simulink model "Pacemaker_group11_requirementtable"  (R2022a)
settings: Solver=FixedStepAuto  StartTime=0.0  StopTime=10.0  FixedStep=1e-3  RelTol=1e-3  EnableMultiTasking=on
undefined symbols (not defined in the file): A0, A1, D0, D1, D10, D11, D12, D13, D2, D3, D4, D5, D6, D7, D8, D9, magnitude, PTA0, PTA1, PTA2, PTB2, PTB23, PTB3, PTB9, PTC16, PTC17, PTC2, PTC3, PTC4, PTD0, PTD1, PTD2, PTD3
libraries: frdmk64flib x20, etargetslib x17, dspstat3 x1, simulink x1
(part 1 of 2)
settings Model: ExtModeTrigDuration=5  Creator=39200  LastModifiedBy=39200
settings OptimizationCC: EnhancedBackFolding=on  PassReuseOutputArgsAs=Individual arguments  ZeroExternalMemoryAtStartup=off  ZeroInternalMemoryAtStartup=off  MaxStackSize=64  OptimizeBlockOrder=speed  DifferentSizesBufferReuse=on  OptimizationCustomize=off  EfficientTunableParamExpr=on
settings DebuggingCC: ParameterTunabilityLossMsg=error
settings HardwareCC: ProdBitPerPointer=32  ProdBitPerSizeT=32  ProdBitPerPtrDiffT=32  ProdLargestAtomicInteger=Long  ProdLargestAtomicFloat=Double  ProdWordSize=32  ProdHWDeviceType=ARM Compatible->ARM Cortex
settings SFSimCC: MATLABDynamicMemAlloc=off
settings RTWCC: SystemTargetFile=ert.tlc  HardwareBoard=NXP FRDM-K64F  TLCOptions="-aInlineSetEventsForThisBaseRateFcn=TLC_FALSE -aSuppressMultiTaskScheduler=TLC_FALSE  -aRateBasedStepFcn=0"  TemplateMakefile=ert_default_tmf  Toolchain=GNU Tools for ARM Embedded Processors
settings CodeAppCC: ForceParamTrailComments=on  IgnoreCustomStorageClasses=off  OperatorAnnotations=on  SimulinkDataObjDesc=on  SFDataObjDesc=on  InsertBlockDesc=on
settings ERTTargetCC: ExtModeTransport=4  ExtModeMexFile=sendToCommService

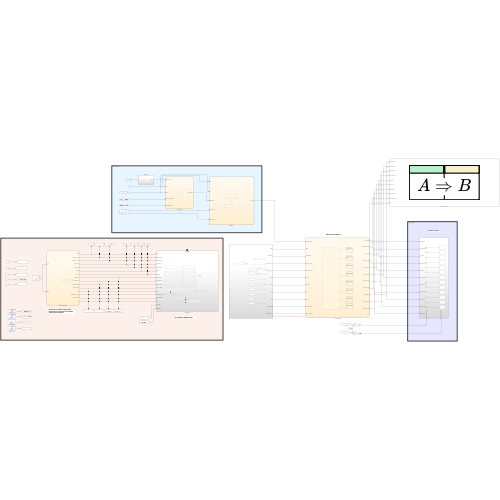
[thumbnail: Simulink's stored preview of the top-level diagram]
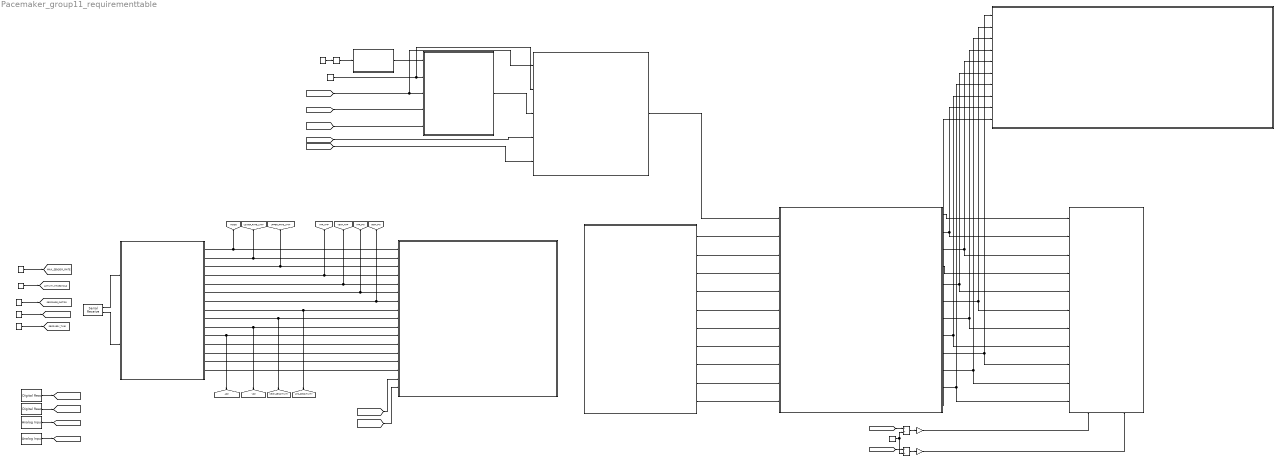
== system Pacemaker_group11_requirementtable ==
  note: Hardware Output
  note: Stateflow for All Modes
  note: Rate Modulation
  note: Stateflow for Initial Programmable Parameters and Input Programmable Parameters from DCM
  note: Inputs
  note: Send Data to DCM through UART
  note: Hardware Output
  ATR_SIGNAL : frdmk64flib/Analog Input  Whichpin=PTB2 (A0)  SampleTime=-1
  Acceleration1 : Subsystem
  Compare To Constant2 : simulink/Logic and Bit Operations/Compare To Constant  relop=>=  const=5  OutDataTypeStr=boolean
  Constant : Constant  Value=3.3
  Constant10 : Constant  Value=5
  Constant11 : Constant  Value=8
  Constant12 : Constant  Value=5
  Constant6 : Constant  Value=60
  Constant7 : Constant  Value=30
  Constant8 : Constant  Value=0.01
  Constant9 : Constant  Value=120
  Digital Read : frdmk64flib/Digital Read  Whichpin=PTC17 (D1)  SampleTime=-1
  Digital Read1 : frdmk64flib/Digital Read  Whichpin=PTC16 (D0)  SampleTime=-1
  Divide2 : Product  Inputs=*/
  Divide3 : Product  Inputs=*/
  Gain : Gain  Gain=100
  Gain1 : Gain  Gain=100
  Requirements Table : Requirements Table  TreatAsAtomicUnit=on
  Serial Communication1 : Stateflow chart  TreatAsAtomicUnit=on
      settings: PortSchema="{\"entries\":[{\"content\":{\"sides\":[{\"content\":{\"connectorIds\":[\"In1\",\"In2\"]},\"type\":\"ConnectorPlacement.EquallySpacedRectSide\",\"uuid\":\"901574a5-7e09-4852-8827-baac8e876273\"},{\"content\":{\"connectorIds\":[\"Out1\",\"Out2\",\"Out3\",\"Out4\",\"Out12\",\"Out5\",\"Out13\",\"Out14\",\"Out10\",\"Out6\",\"Out11\",\"Out7\",\"Out9\",\"Out8\",\"Out15\"],\"side\":\"RIGHT\"},\"type\":\"ConnectorPlacement.EquallySpacedRectSide\",\"uuid\":\"89d36c37-e833-4dfe-ae0b-2d9eccbce05b\"},{\"content\":{\"connectorIds\":[],\"side\":\"TOP\"},\"type\":\"ConnectorPlacement.EquallySpacedRectSide\",\"uuid\":\"eeb52db1-ccd5-49db-acea-74a4d3271ab8\"}]},\"type\":\"ConnectorPlacement.EquallySpacedConnector\",\"uuid\":\"16ccc146-147c-46a9-b907-deab62e4a6a6\"}],\"packageUris\":[\"http://schema.mathworks.com/mf0/Connector/R2020b\"],\"version\":\"1.0\"}"
  Serial Receive : frdmk64flib/Serial Receive  SCIModule=0  Baudrate=uint32(9600)  Parity=None  StopBits=1  HardwareFlowControl=None  ByteOrder=LittleEndian  DataType=uint8  DataLength=66  BlockingMode=off  OutputStatus=on  SampleTime=-1
  Serial transmit : Subsystem  TreatAsAtomicUnit=on
  Subsystem : Subsystem
      settings: PortSchema="{\"entries\":[{\"content\":{\"sides\":[{\"content\":{\"connectorIds\":[\"In1\",\"In2\",\"In3\",\"In4\",\"In5\",\"In6\",\"In7\",\"In8\",\"In9\",\"In10\",\"In11\"]},\"type\":\"ConnectorPlacement.EquallySpacedRectSide\",\"uuid\":\"cf431d19-a261-4061-b975-82ab8e4554ba\"},{\"content\":{\"connectorIds\":[],\"side\":\"RIGHT\"},\"type\":\"ConnectorPlacement.EquallySpacedRectSide\",\"uuid\":\"d9d96e0a-6018-4f8e-a98f-6eed3a91414e\"},{\"content\":{\"connectorIds\":[],\"side\":\"TOP\"},\"type\":\"ConnectorPlacement.EquallySpacedRectSide\",\"uuid\":\"2358aaff-c3a0-4959-bedb-835f64f1bbed\"},{\"content\":{\"connectorIds\":[\"In12\",\"In13\"],\"side\":\"BOTTOM\"},\"type\":\"ConnectorPlacement.EquallySpacedRectSide\",\"uuid\":\"ece4eb5b-308d-4002-b014-99ad51b61e06\"}]},\"type\":\"ConnectorPlacement.EquallySpacedConnector\",\"uuid\":\"cdbd5127-fb13-4f48-9ecc-e21d40fbaa52\"}],\"packageUris\":[\"http://schema.mathworks.com/mf0/Connector/R2020b\"],\"version\":\"1.0\"}"
  Subsystem1 : Subsystem
  VENT_SIGNAL : frdmk64flib/Analog Input  Whichpin=PTB3 (A1)  SampleTime=-1
  eight model stateflow : Stateflow chart  TreatAsAtomicUnit=on
      settings: PortSchema="{\"entries\":[{\"content\":{\"sides\":[{\"content\":{\"connectorIds\":[\"In6\",\"In7\",\"In2\",\"In4\",\"In1\",\"In8\",\"In9\",\"In11\",\"In10\",\"In5\",\"In3\"]},\"type\":\"ConnectorPlacement.EquallySpacedRectSide\",\"uuid\":\"7bd189cb-d286-447b-b347-38d7b12e59ee\"},{\"content\":{\"connectorIds\":[\"Out1\",\"Out2\",\"Out3\",\"Out4\",\"Out5\",\"Out6\",\"Out7\",\"Out8\",\"Out9\",\"Out10\",\"Out11\",\"Out12\"],\"side\":\"RIGHT\"},\"type\":\"ConnectorPlacement.EquallySpacedRectSide\",\"uuid\":\"522f4543-8a7d-441b-9c0c-141bccf5cf26\"},{\"content\":{\"connectorIds\":[],\"side\":\"TOP\"},\"type\":\"ConnectorPlacement.EquallySpacedRectSide\",\"uuid\":\"cf7ae06b-6ef3-498b-825a-38a0a4c90c8a\"}]},\"type\":\"ConnectorPlacement.EquallySpacedConnector\",\"uuid\":\"ae15f7ff-4998-48cc-acd9-270deb6c013f\"}],\"packageUris\":[\"http://schema.mathworks.com/mf0/Connector/R2020b\"],\"version\":\"1.0\"}"
  get desired rate : Stateflow chart  TreatAsAtomicUnit=on
  get target rate : Stateflow chart  TreatAsAtomicUnit=on
      settings: PortSchema="{\"entries\":[{\"content\":{\"sides\":[{\"content\":{\"connectorIds\":[\"In3\",\"In2\",\"In1\",\"In4\",\"In5\"]},\"type\":\"ConnectorPlacement.EquallySpacedRectSide\",\"uuid\":\"b1115713-3752-47d5-be72-104b51cdb1c5\"},{\"content\":{\"connectorIds\":[\"Out1\"],\"side\":\"RIGHT\"},\"type\":\"ConnectorPlacement.EquallySpacedRectSide\",\"uuid\":\"0930a30a-8aa5-4912-ba1f-cc7f148656b0\"},{\"content\":{\"connectorIds\":[],\"side\":\"TOP\"},\"type\":\"ConnectorPlacement.EquallySpacedRectSide\",\"uuid\":\"94dfeeb6-c083-4dc2-b4f5-32fe99d16bb7\"}]},\"type\":\"ConnectorPlacement.EquallySpacedConnector\",\"uuid\":\"5d93a560-4d98-406a-ad12-5273aac4a25c\"}],\"packageUris\":[\"http://schema.mathworks.com/mf0/Connector/R2020b\"],\"version\":\"1.0\"}"
  tag scope: ACTIVITY_THRESHOLD=global, ARP=global, ATR_AMP=global, ATR_CMP_DETECT=global, ATR_PW=global, ATR_SENSITIVITY=global, ATR_SIGNAL=global, LOWER_RATE_LIMIT=global, MAX_SENSOR_RATE=global, MODE=global, REACTION_TIME=global, RECOVERY_TIME=global, RESPONSE_FACTOR=global, UPPER_RATE_LIMIT=global, VENT_AMP=global, VENT_CMP_DETECT=global, VENT_PW=global, VENT_SENSITIVITY=global, VENT_SIGNAL=global, VRP=global
  wires:
  Subsystem1/8(VRP) -> eight model stateflow/10(VRP)
  [RECOVERY_TIME] -> get target rate/5(RECOVER_TIME)
  Digital Read/1 -> [VENT_CMP_DETECT]
  Serial Communication1/15(Type) -> Serial transmit/15(Type)
  ATR_SIGNAL/1 -> [ATR_SIGNAL]
  Digital Read1/1 -> [ATR_CMP_DETECT]
  Subsystem1/7(ARP) -> eight model stateflow/11(ARP)
  VENT_SIGNAL/1 -> [VENT_SIGNAL]
  [VENT_SIGNAL] -> Serial transmit/17(VENT_SIGNAL)
  Constant7/1 -> [REACTION_TIME]
  Serial Receive/2 -> Serial Communication1/2(status)
  Serial Communication1/6(VENT_REF_PERIOD) -> Serial transmit/10(VENT_REF_PERIOD), [VRP]
  eight model stateflow/7(VENT_PACE_CTRL) -> Subsystem/7(VENT_PACE_CTRL), Requirements Table/4(VENT_PACE_CTRL)
  Subsystem1/1(MODE) -> eight model stateflow/7(MODE)
  Gain1/1 -> Subsystem/12(ATR_CMP_REF_PWM)
  Divide2/1 -> Gain/1
  Subsystem1/9(ATR_CMP_DETECT) -> eight model stateflow/5(ATR_CMP_DETECT)
  Serial Communication1/7(PVARP) -> Serial transmit/12(PVARP)
  Serial Communication1/9(HYSTERESIS_RATE_LIMIT) -> Serial transmit/13(HYSTERESIS_RATE_LIMIT)
  Divide3/1 -> Gain1/1
  Subsystem1/5(ATR_PW) -> eight model stateflow/8(ATR_PW)
  Serial Communication1/13(VENT_PW) -> [VENT_PW], Serial transmit/7(VENT_PW)
  Subsystem1/10(VENT_CMP_DETECT) -> eight model stateflow/3(VENT_CMP_DETECT)
  eight model stateflow/5(Z_VENT_CTRL) -> Subsystem/5(Z_VENT_CTRL), Requirements Table/6(Z_VENT_CTRL)
  Subsystem1/2(PULSE_PERIOD) -> eight model stateflow/2(PULSE_PERIOD)
  eight model stateflow/3(Z_ATR_CTRL) -> Subsystem/3(Z_ATR_CTRL), Requirements Table/5(Z_ATR_CTRL)
  eight model stateflow/4(PACING_REF_PWM) -> Subsystem/4(PACING_REF_PWM)
  eight model stateflow/2(PACE_CHARGE_CTRL) -> Subsystem/2(PACE_CHARGE_CTRL), Requirements Table/9(PACE_CHARGE_CTRL)
  eight model stateflow/1(IS_CHARGING) -> Subsystem/1(IS_CHARGING)
  Serial Communication1/3(UPPER_RATE_LIMIT) -> [UPPER_RATE_LIMIT], Serial transmit/3(UPPER_RATE_LIMIT)
  [VENT_SENSITIVITY] -> Divide2/1
  [ATR_SIGNAL] -> Serial transmit/16(ATR_SIGNAL)
  Serial Communication1/11(ATR_REF_PERIOD) -> [ARP], Serial transmit/11(ATR_REF_PERIOD)
  Serial Communication1/2(LOWER_RATE_LIMIT) -> [LOWER_RATE_LIMIT], Serial transmit/2(LOWER_RATE_LIMIT)
  [ATR_SENSITIVITY] -> Divide3/1
  Serial Receive/1 -> Serial Communication1/1(rxdata)
  Serial Communication1/5(ATR_PW) -> [ATR_PW], Serial transmit/6(ATR_PW)
  Subsystem1/6(VENT_PW) -> eight model stateflow/9(VENT_PW)
  Subsystem1/4(VENT_DUTY_CYCLE) -> eight model stateflow/1(VENT_DUTY_CYCLE)
  Compare To Constant2/1 -> Acceleration1/1(In1)
  get desired rate/1(DESIRED_RATE) -> get target rate/1(DESIRED_RATE)
  eight model stateflow/6(ATR_PACE_CTRL) -> Subsystem/6(ATR_PACE_CTRL), Requirements Table/2(ATR_PACE_CTRL)
  Constant12/1 -> Compare To Constant2/1
  Serial Communication1/12(VENT_AMP_REG) -> Serial transmit/5(VENT_AMP_REG), [VENT_AMP]
  Serial Communication1/10(VENT_SENSITIVITY) -> Serial transmit/9(VENT_SENSITIVITY), [VENT_SENSITIVITY]
  Constant/1 -> Divide2/2, Divide3/2
  eight model stateflow/8(PACE_GND_CTRL) -> Subsystem/8(PACE_GND_CTRL), Requirements Table/8(PACE_GND_CTRL)
  eight model stateflow/9(ATR_GND_CTRL) -> Subsystem/9(ATR_GND_CTRL), Requirements Table/1(ATR_GND_CTRL)
  Serial Communication1/4(ATR_AMP_REG) -> Serial transmit/4(ATR_AMP_REG), [ATR_AMP]
  Serial Communication1/8(RATE_SMOOTHING) -> Serial transmit/14(RATE_SMOOTHING)
  [REACTION_TIME] -> get target rate/4(REACTION_TIME)
  Serial Communication1/14(ATR_SENSITIVITY) -> [ATR_SENSITIVITY], Serial transmit/8(ATR_SENSITIVITY)
  Acceleration1/1(ACTIVITY) -> get desired rate/1(ACTIVITY_LEVEL)
  [MAX_SENSOR_RATE] -> get desired rate/3(MSR), get target rate/3(MSR)
  eight model stateflow/11(FRONTEND_CTRL) -> Subsystem/11(FRONTEND_CTRL), Requirements Table/7(FRONTEND_CTRL)
  Constant8/1 -> [ACTIVITY_THRESHOLD]
  Constant11/1 -> [RESPONSE_FACTOR]
  eight model stateflow/10(VENT_GND_CTRL) -> Subsystem/10(VENT_GND_CTRL), Requirements Table/3(VENT_GND_CTRL)
  Constant9/1 -> [MAX_SENSOR_RATE]
  [ACTIVITY_THRESHOLD] -> get desired rate/4(ACTIVITY_THRESHOLD)
  Gain/1 -> Subsystem/13(VENT_CMP_REF_PWM)
  Constant10/1 -> [RECOVERY_TIME]
  Constant6/1 -> get desired rate/2(LRL), get target rate/2(LRL)
  Subsystem1/3(ATR_DUTY_CYCLE) -> eight model stateflow/4(ATR_DUTY_CYCLE)
  get target rate/1(Target_rate) -> eight model stateflow/6(MODIFIED_PERIOD)
  Serial Communication1/1(MODE) -> [MODE], Serial transmit/1(MODE)
  ? -> ?
  [RESPONSE_FACTOR] -> get desired rate/5(RESPONSE_FACTOR)
  eight model stateflow/12(status) -> Requirements Table/10(status)

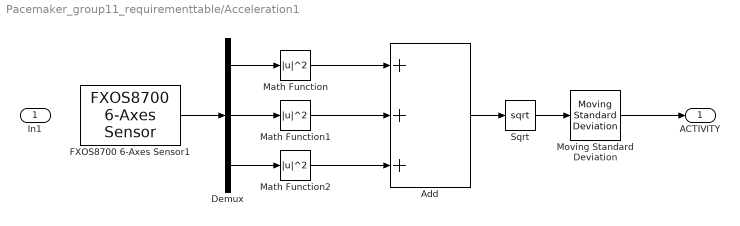
== system Pacemaker_group11_requirementtable/Acceleration1 ==
  In1 : Inport
  Add : Sum  Inputs=+++
  Demux : Demux  Outputs=3
  FXOS8700 6-Axes Sensor1 : frdmk64flib/FXOS8700 6-Axes Sensor  Activesensor=Accelerometer only  ODR=800Hz  HybridODR=400Hz  Accelfullrange=-4g to +4g  SampleTime=-1
  Math Function : Math  Operator=magnitude^2  SignedPower=on  OutDataTypeStr=double
  Math Function1 : Math  Operator=magnitude^2  SignedPower=on  OutDataTypeStr=double
  Math Function2 : Math  Operator=magnitude^2  SignedPower=on  OutDataTypeStr=double
  Moving Standard Deviation : dspstat3/Moving Standard Deviation  Method=Sliding window  ForgettingFactorPort=off  SpecifyWindowLength=on  WindowLength=4  ForgettingFactor=0.9  SimulateUsing=Code generation
      settings: SourceProductBaseCode=DS
  Sqrt : Sqrt
  ACTIVITY : Outport  SourceOfInitialOutputValue=Input signal
  wires:
  Sqrt/1 -> Moving Standard Deviation/1
  Math Function2/1 -> Add/3
  Add/1 -> Sqrt/1
  Math Function1/1 -> Add/2
  Demux/1 -> Math Function/1
  Demux/2 -> Math Function1/1
  Math Function/1 -> Add/1
  FXOS8700 6-Axes Sensor1/1 -> Demux/1
  Demux/3 -> Math Function2/1
  Moving Standard Deviation/1 -> ACTIVITY/1

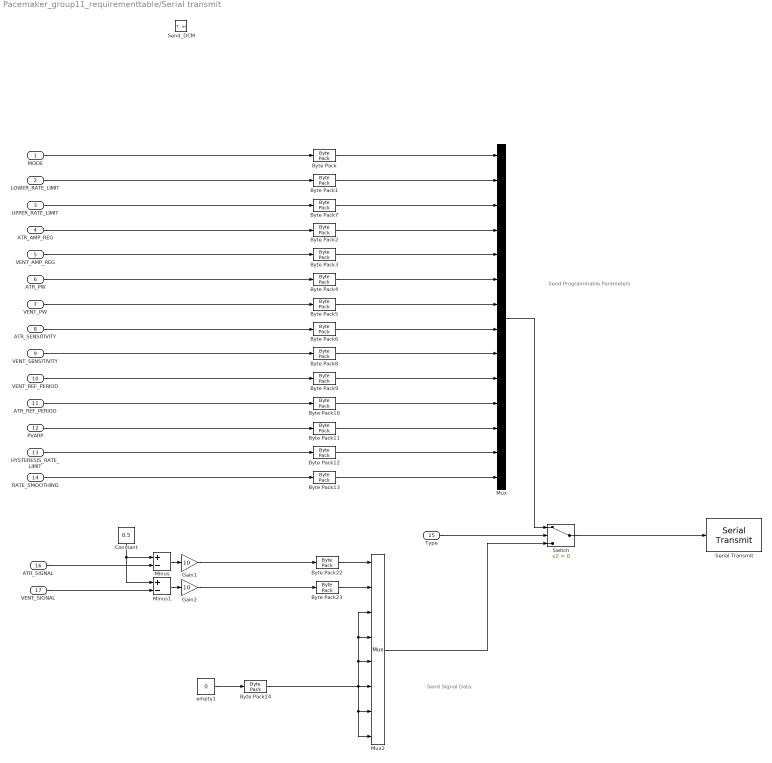
== system Pacemaker_group11_requirementtable/Serial transmit ==
  note: Send Signal Data
  note: Send Programmable Parameters
  MODE : Inport
  LOWER_RATE_LIMIT : Inport  Port=2
  UPPER_RATE_LIMIT : Inport  Port=3
  ATR_AMP_REG : Inport  Port=4
  VENT_AMP_REG : Inport  Port=5
  ATR_PW : Inport  Port=6
  VENT_PW : Inport  Port=7
  ATR_SENSITIVITY : Inport  Port=8
  VENT_SENSITIVITY : Inport  Port=9
  VENT_REF_PERIOD : Inport  Port=10
  ATR_REF_PERIOD : Inport  Port=11
  PVARP : Inport  Port=12
  HYSTERESIS_RATE_LIMIT : Inport  Port=13
  RATE_SMOOTHING : Inport  Port=14
  Type : Inport  Port=15
  ATR_SIGNAL : Inport  Port=16
  VENT_SIGNAL : Inport  Port=17
  Send_DCM : TriggerPort  TriggerType=function-call  IsSimulinkFunction=on  FunctionName=Send_DCM  VariantControl=Variant
  Byte Pack{,1,7,9..13} (8 alike) : etargetslib/Byte Pack  datatypes={'uint16'}  byteAlign=1
  Byte Pack{2..6,8,22..24} (9 alike) : etargetslib/Byte Pack  datatypes={'double'}  byteAlign=1
  Constant : Constant  Value=0.5
  Gain1 : Gain  Gain=10
  Gain2 : Gain  Gain=10
  Minus : Sum  Inputs=+-
  Minus1 : Sum  Inputs=+-
  Mux : Mux  Inputs=14
  Mux2 : Mux  Inputs=8
  Serial Transmit : frdmk64flib/Serial Transmit  SCIModule=0  Baudrate=uint32(9600)  Parity=None  StopBits=1  HardwareFlowControl=None  ByteOrder=LittleEndian  BlockingMode=on  OutputStatus=off
  Switch : Switch  Criteria=u2 > Threshold  SaturateOnIntegerOverflow=off  InputSameDT=off
  empty1 : Constant  Value=0
  wires:
  MODE/1 -> Byte Pack/1
  LOWER_RATE_LIMIT/1 -> Byte Pack1/1
  UPPER_RATE_LIMIT/1 -> Byte Pack7/1
  ATR_AMP_REG/1 -> Byte Pack2/1
  VENT_AMP_REG/1 -> Byte Pack3/1
  ATR_PW/1 -> Byte Pack4/1
  VENT_PW/1 -> Byte Pack5/1
  VENT_SENSITIVITY/1 -> Byte Pack8/1
  ATR_SENSITIVITY/1 -> Byte Pack6/1
  RATE_SMOOTHING/1 -> Byte Pack13/1
  HYSTERESIS_RATE_LIMIT/1 -> Byte Pack12/1
  PVARP/1 -> Byte Pack11/1
  ATR_REF_PERIOD/1 -> Byte Pack10/1
  VENT_REF_PERIOD/1 -> Byte Pack9/1
  Byte Pack1/1 -> Mux/2
  Byte Pack7/1 -> Mux/3
  Byte Pack/1 -> Mux/1
  Byte Pack2/1 -> Mux/4
  Byte Pack3/1 -> Mux/5
  Byte Pack4/1 -> Mux/6
  Byte Pack5/1 -> Mux/7
  Byte Pack6/1 -> Mux/8
  Byte Pack8/1 -> Mux/9
  Byte Pack9/1 -> Mux/10
  Byte Pack10/1 -> Mux/11
  Byte Pack11/1 -> Mux/12
  Byte Pack12/1 -> Mux/13
  Byte Pack13/1 -> Mux/14
  Type/1 -> Switch/2
  Mux/1 -> Switch/1
  Switch/1 -> Serial Transmit/1
  Minus/1 -> Gain1/1
  ATR_SIGNAL/1 -> Minus/2
  Constant/1 -> Minus1/1, Minus/1
  Minus1/1 -> Gain2/1
  VENT_SIGNAL/1 -> Minus1/2
  Gain1/1 -> Byte Pack22/1
  Byte Pack23/1 -> Mux2/2
  Byte Pack24/1 -> Mux2/8, Mux2/7, Mux2/6, Mux2/5, Mux2/3, Mux2/4
  empty1/1 -> Byte Pack24/1
  Mux2/1 -> Switch/3
  Gain2/1 -> Byte Pack23/1
  Byte Pack22/1 -> Mux2/1

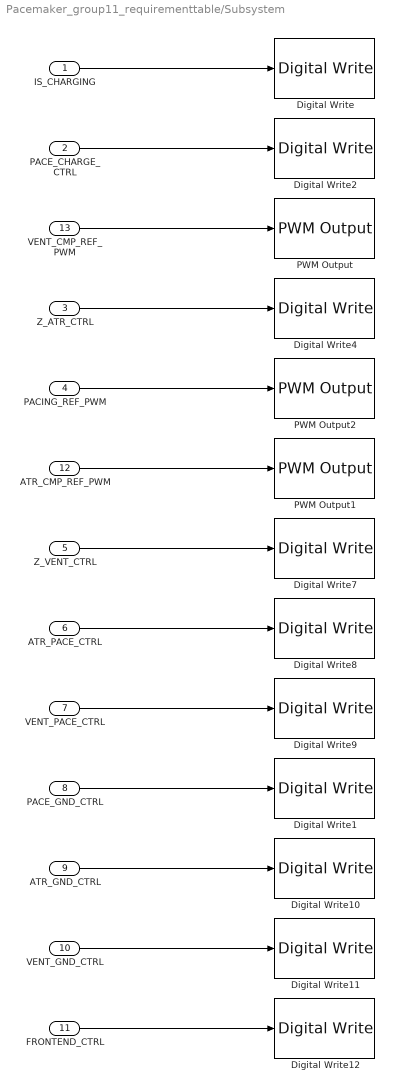
== system Pacemaker_group11_requirementtable/Subsystem ==
  IS_CHARGING : Inport
  PACE_CHARGE_CTRL : Inport  Port=2
  Z_ATR_CTRL : Inport  Port=3
  PACING_REF_PWM : Inport  Port=4
  Z_VENT_CTRL : Inport  Port=5
  ATR_PACE_CTRL : Inport  Port=6
  VENT_PACE_CTRL : Inport  Port=7
  PACE_GND_CTRL : Inport  Port=8
  ATR_GND_CTRL : Inport  Port=9
  VENT_GND_CTRL : Inport  Port=10
  FRONTEND_CTRL : Inport  Port=11
  ATR_CMP_REF_PWM : Inport  Port=12
  VENT_CMP_REF_PWM : Inport  Port=13
  Digital Write : frdmk64flib/Digital Write  Whichpin=RED_LED
  Digital Write1 : frdmk64flib/Digital Write  Whichpin=PTD0 (D10)
  Digital Write10 : frdmk64flib/Digital Write  Whichpin=PTD2 (D11)
  Digital Write11 : frdmk64flib/Digital Write  Whichpin=PTD3 (D12)
  Digital Write12 : frdmk64flib/Digital Write  Whichpin=PTD1 (D13)
  Digital Write2 : frdmk64flib/Digital Write  Whichpin=PTB9 (D2)
  Digital Write4 : frdmk64flib/Digital Write  Whichpin=PTB23 (D4)
  Digital Write7 : frdmk64flib/Digital Write  Whichpin=PTC3 (D7)
  Digital Write8 : frdmk64flib/Digital Write  Whichpin=PTA0 (D8)
  Digital Write9 : frdmk64flib/Digital Write  Whichpin=PTC4 (D9)
  PWM Output : frdmk64flib/PWM Output  Whichpin=PTA1 (D3)  InitialFrequency=2000  InitialDutyCycle=0
  PWM Output1 : frdmk64flib/PWM Output  Whichpin=PTC2 (D6)  InitialFrequency=2000  InitialDutyCycle=0
  PWM Output2 : frdmk64flib/PWM Output  Whichpin=PTA2 (D5)  InitialFrequency=2000  InitialDutyCycle=0
  wires:
  PACE_GND_CTRL/1 -> Digital Write1/1
  Z_ATR_CTRL/1 -> Digital Write4/1
  IS_CHARGING/1 -> Digital Write/1
  PACE_CHARGE_CTRL/1 -> Digital Write2/1
  ATR_PACE_CTRL/1 -> Digital Write8/1
  Z_VENT_CTRL/1 -> Digital Write7/1
  VENT_PACE_CTRL/1 -> Digital Write9/1
  ATR_GND_CTRL/1 -> Digital Write10/1
  PACING_REF_PWM/1 -> PWM Output2/1
  VENT_CMP_REF_PWM/1 -> PWM Output/1
  ATR_CMP_REF_PWM/1 -> PWM Output1/1
  FRONTEND_CTRL/1 -> Digital Write12/1
  VENT_GND_CTRL/1 -> Digital Write11/1

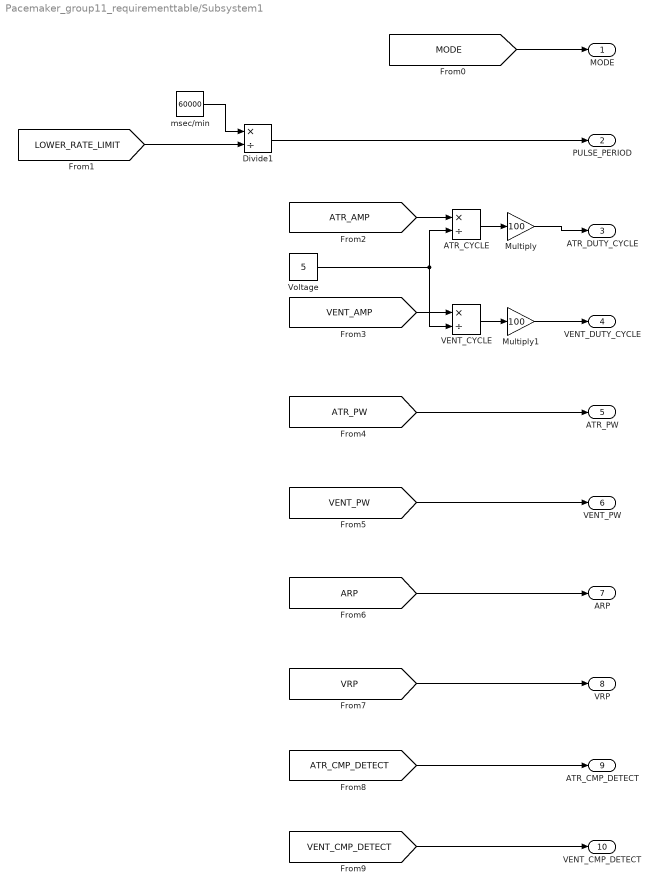
== system Pacemaker_group11_requirementtable/Subsystem1 ==
  ATR_CYCLE : Product  Inputs=*/
  Divide1 : Product  Inputs=*/
  Multiply : Gain  Gain=100
  Multiply1 : Gain  Gain=100
  VENT_CYCLE : Product  Inputs=*/
  Voltage : Constant  Value=5
  msec/min : Constant  Value=60000  OutDataTypeStr=double  LockScale=on
  MODE : Outport
  PULSE_PERIOD : Outport  Port=2
  ATR_DUTY_CYCLE : Outport  Port=3
  VENT_DUTY_CYCLE : Outport  Port=4
  ATR_PW : Outport  Port=5
  VENT_PW : Outport  Port=6
  ARP : Outport  Port=7
  VRP : Outport  Port=8
  ATR_CMP_DETECT : Outport  Port=9
  VENT_CMP_DETECT : Outport  Port=10
  wires:
  msec/min/1 -> Divide1/1
  [LOWER_RATE_LIMIT] -> Divide1/2
  Divide1/1 -> PULSE_PERIOD/1
  Voltage/1 -> VENT_CYCLE/2, ATR_CYCLE/2
  ATR_CYCLE/1 -> Multiply/1
  VENT_CYCLE/1 -> Multiply1/1
  [MODE] -> MODE/1
  Multiply1/1 -> VENT_DUTY_CYCLE/1
  Multiply/1 -> ATR_DUTY_CYCLE/1
  [ATR_AMP] -> ATR_CYCLE/1
  [VENT_AMP] -> VENT_CYCLE/1
  [ATR_PW] -> ATR_PW/1
  [VENT_PW] -> VENT_PW/1
  [ARP] -> ARP/1
  [VRP] -> VRP/1
  [ATR_CMP_DETECT] -> ATR_CMP_DETECT/1
  [VENT_CMP_DETECT] -> VENT_CMP_DETECT/1

== stateflow chart Pacemaker_group11_requirementtable/Serial Communication1 ==
  state SettingParameters
    entry:
    MODE = typecast(rxdata(3:4), 'uint16');
    LOWER_RATE_LIMIT = typecast(rxdata(5:6), 'uint16'); % ppm
    UPPER_RATE_LIMIT = typecast(rxdata(7:8), 'uint16'); % ppm
    ATR_AMP_REG =  typecast(rxdata(9:16), 'double'); % V
    VENT_AMP_REG = typecast(rxdata(17:24), 'double'); % V
    ATR_PW = typecast(rxdata(25:32), 'double'); % ms
    VENT_PW = typecast(rxdata(33:40), 'double'); % ms
    ATR_SENSITIVITY = typecast(rxdata(41:48), 'double'); % mV
    VENT_SENSITIVITY = typecast(rxdata(49:56), 'double'); % mV
    ATR_REF_PERIOD = typecast(rxdata(57:58), 'uint16'); % ms
    VENT_REF_PERIOD = typecast(rxdata(59:60), 'uint16'); % ms
    PVARP = typecast(rxdata(61:62), 'uint16'); % ms
    HYSTERESIS_RATE_LIMIT = typecast(rxdata(63:64), 'uint16'); % ms
    RATE_SMOOTHING = typecast(rxdata(65:66), 'uint16'); % percentage
  state Init
    entry:
    MODE = 0;
    LOWER_RATE_LIMIT = 60;
    UPPER_RATE_LIMIT = 120;
    %MAX_SENSOR_RATE = typecast(rxdata(7:8), 'uint16'); % ppm
    %FIXED_AV_DELAY = typecast(rxdata(9:10), 'uint16'); % ms
    %DYNAMIC_AV_DELAY = rxdata(11); % boolean
    %MIN_DYNAMIC_AV_DELAY =  typecast(rxdata(12:13), 'uint16'); % ms
    %SENSED_AV_DELAY_OFFSET = typecast(rxdata(14:15), 'uint16'); % ms
    ATR_AMP_REG =  3.5; % V
    VENT_AMP_REG = 3.5; % V
    %ATR_AMP_UNREG = typecast(rxdata(9:16), 'double'); % V
    %VENT_AMP_UNREG = typecast(rxdata(9:16), 'double'); % V
    ATR_PW = 0.4; % ms
    VENT_PW = 0.4; % ms
    ATR_SENSITIVITY = 0.75; % mV
    VENT_SENSITIVITY = 2.5; % mV
    ATR_REF_PERIOD = 250; % ms
    VENT_REF_PERIOD = 320; % ms
    PVARP = 250; % ms
    %PVARP_EXTENSION = typecast(rxdata(14:15), 'uint16'); % ms
    HYSTERESIS_RATE_LIMIT = 0; % ms
    RATE_SMOOTHING = 0; % percentage
  state STANDBY
    %Waiting for COM
  state ECHO_PARAM1
    entry:
    Type = 0
    Send_DCM();
  state ECHO_PARAM
    entry:
    Type = 1
    Send_DCM();
  (default) -> Init
  SettingParameters -> STANDBY
  (junction 96) -> STANDBY [order 2]
  (junction 94) -> SettingParameters [order 3] : [rxdata(2) == hex2dec('55')]
  STANDBY -> (junction 96) : [status == 0]
  (junction 96) -> (junction 94) [order 1] : [rxdata(1) == hex2dec('16')]
  Init -> STANDBY
  (junction 94) -> ECHO_PARAM [order 1] : [rxdata(2) == hex2dec('22')]
  (junction 94) -> ECHO_PARAM1 [order 2] : [rxdata(2) == hex2dec('33')]
  ECHO_PARAM -> STANDBY
  ECHO_PARAM1 -> STANDBY
  data: MODE output uint16; LOWER_RATE_LIMIT output uint16; UPPER_RATE_LIMIT output uint16; ATR_AMP_REG output double; ATR_PW output double; rxdata input uint8; status input uint8; VENT_REF_PERIOD output uint16; PVARP output uint16; RATE_SMOOTHING output uint16; HYSTERESIS_RATE_LIMIT output uint16; VENT_SENSITIVITY output double; ATR_REF_PERIOD output uint16; VENT_AMP_REG output double; VENT_PW output double; ATR_SENSITIVITY output; Type output

== stateflow chart Pacemaker_group11_requirementtable/Requirements Table ==
  (default) -> (junction 1073741860)
  (junction 1073741860) -> (junction 1073741861) : {
      | % SF_REQ_REV_07
      | }
  (junction 1073741861) -> (junction 1073741863) : {
      | % HEADER_ASSIGNMENTS
      |
      | }
  (junction 1073741863) -> (junction 1073741865) : {
      | % START_A_4
      | }
  (junction 1073741865) -> (junction 1073741867) : {
      | }
  (junction 1073741867) -> (junction 1073741869)
  (junction 1073741869) -> (junction 1073741871) : {
      | }
  (junction 1073741871) -> (junction 1073741873) : {
      | % END_A_4
      | }
  (junction 1073741873) -> (junction 1073741910) : {
      | % START_R_1
      | }
  (junction 1073741910) -> (junction 1073741912) : {
      | }
  (junction 1073741912) -> (junction 1073741914) : {
      |
      |
      | }
  (junction 1073741914) -> (junction 1073741916) : {
      | }
  (junction 1073741916) -> (junction 1073741944) : {
      | % START_R_7
      | }
  (junction 1073741944) -> (junction 1073741946) : {
      | }
  (junction 1073741946) -> (junction 1073741948)
  (junction 1073741948) -> (junction 1073741950) [order 1] : [(((status) == (00000)))]
  (junction 1073741948) -> (junction 1073741956) [order 2]
  (junction 1073741950) -> (junction 1073741952) : {
      | reqtable_postcondition((((PACE_CHARGE_CTRL) == (1))) && (((Z_ATR_CTRL) == (0))) && (((Z_VENT_CTRL) == (0))) && (((ATR_PACE_CTRL) == (0))) && (((VENT_PACE_CTRL) == (0))) && (((PACE_GND_CTRL) == (1))) && (((ATR_GND_CTRL) == (1))) && (((VENT_GND_CTRL) == (0))) && (((FRONTEND_CTRL) == (0))), 'R:1.1');
      |
      |
      | }
  (junction 1073741952) -> (junction 1073741954) : {
      | }
  (junction 1073741954) -> (junction 1073741956)
  (junction 1073741956) -> (junction 1073741958)
  (junction 1073741958) -> (junction 1073741960) : {
      | % END_R_7
      | }
  (junction 1073741960) -> (junction 1073741965) : {
      | % START_R_10
      | }
  (junction 1073741965) -> (junction 1073741967) : {
      | }
  (junction 1073741967) -> (junction 1073741969)
  (junction 1073741969) -> (junction 1073741971) [order 1] : [(((status) == (00001)))]
  (junction 1073741969) -> (junction 1073741977) [order 2]
  (junction 1073741971) -> (junction 1073741973) : {
      | reqtable_postcondition((((PACE_CHARGE_CTRL) == (0))) && (((Z_ATR_CTRL) == (0))) && (((Z_VENT_CTRL) == (0))) && (((ATR_PACE_CTRL) == (1))) && (((VENT_PACE_CTRL) == (0))) && (((PACE_GND_CTRL) == (1))) && (((ATR_GND_CTRL) == (0))) && (((VENT_GND_CTRL) == (0))) && (((FRONTEND_CTRL) == (0))), 'R:1.2');
      |
      |
      | }
  (junction 1073741973) -> (junction 1073741975) : {
      | }
  (junction 1073741975) -> (junction 1073741977)
  (junction 1073741977) -> (junction 1073741979)
  (junction 1073741979) -> (junction 1073741981) : {
      | % END_R_10
      | }
  (junction 1073741981) -> (junction 1073741928) : {
      | % END_R_1
      | }
  (junction 1073741928) -> (junction 1073741998) : {
      | % START_R_13
      | }
  (junction 1073741998) -> (junction 1073742000) : {
      | }
  (junction 1073742000) -> (junction 1073742002) : {
      |
      |
      | }
  (junction 1073742002) -> (junction 1073742004) : {
      | }
  (junction 1073742004) -> (junction 1073742032) : {
      | % START_R_16
      | }
  (junction 1073742032) -> (junction 1073742034) : {
      | }
  (junction 1073742034) -> (junction 1073742036)
  (junction 1073742036) -> (junction 1073742038) [order 1] : [(((status) == (00010)))]
  (junction 1073742036) -> (junction 1073742044) [order 2]
  (junction 1073742038) -> (junction 1073742040) : {
      | reqtable_postcondition((((PACE_CHARGE_CTRL) == (1))) && (((Z_ATR_CTRL) == (0))) && (((Z_VENT_CTRL) == (0))) && (((ATR_PACE_CTRL) == (0))) && (((VENT_PACE_CTRL) == (0))) && (((PACE_GND_CTRL) == (1))) && (((ATR_GND_CTRL) == (0))) && (((VENT_GND_CTRL) == (1))) && (((FRONTEND_CTRL) == (0))), 'R:2.1');
      |
      |
      | }
  (junction 1073742040) -> (junction 1073742042) : {
      | }
  (junction 1073742042) -> (junction 1073742044)
  (junction 1073742044) -> (junction 1073742046)
  (junction 1073742046) -> (junction 1073742048) : {
      | % END_R_16
      | }
  (junction 1073742048) -> (junction 1073742053) : {
      | % START_R_19
      | }
  (junction 1073742053) -> (junction 1073742055) : {
      | }
  (junction 1073742055) -> (junction 1073742057)
  (junction 1073742057) -> (junction 1073742059) [order 1] : [(((status) == (00011)))]
  (junction 1073742057) -> (junction 1073742065) [order 2]
  (junction 1073742059) -> (junction 1073742061) : {
      | reqtable_postcondition((((PACE_CHARGE_CTRL) == (0))) && (((Z_ATR_CTRL) == (0))) && (((Z_VENT_CTRL) == (0))) && (((ATR_PACE_CTRL) == (0))) && (((VENT_PACE_CTRL) == (0))) && (((PACE_GND_CTRL) == (1))) && (((ATR_GND_CTRL) == (0))) && (((VENT_GND_CTRL) == (0))) && (((FRONTEND_CTRL) == (0))), 'R:2.2');
      |
      |
      | }
  (junction 1073742061) -> (junction 1073742063) : {
      | }
  (junction 1073742063) -> (junction 1073742065)
  (junction 1073742065) -> (junction 1073742067)
  (junction 1073742067) -> (junction 1073742069) : {
      | % END_R_19
      | }
  (junction 1073742069) -> (junction 1073742016) : {
      | % END_R_13
      | }
  (junction 1073742016) -> (junction 1073742086) : {
      | % START_R_22
      | }
  (junction 1073742086) -> (junction 1073742088) : {
      | }
  (junction 1073742088) -> (junction 1073742090) : {
      |
      |
      | }
  (junction 1073742090) -> (junction 1073742092) : {
      | }
  (junction 1073742092) -> (junction 1073742200) : {
      | % START_R_25
      | }
  (junction 1073742200) -> (junction 1073742202) : {
      | }
  (junction 1073742202) -> (junction 1073742204)
  (junction 1073742204) -> (junction 1073742206) [order 1] : [(((status) == (00100)))]
  (junction 1073742204) -> (junction 1073742212) [order 2]
  (junction 1073742206) -> (junction 1073742208) : {
      | reqtable_postcondition((((PACE_CHARGE_CTRL) == (1))) && (((Z_ATR_CTRL) == (0))) && (((Z_VENT_CTRL) == (0))) && (((ATR_PACE_CTRL) == (0))) && (((VENT_PACE_CTRL) == (0))) && (((PACE_GND_CTRL) == (1))) && (((ATR_GND_CTRL) == (1))) && (((VENT_GND_CTRL) == (0))) && (((FRONTEND_CTRL) == (1))), 'R:3.1');
      |
      |
      | }
  (junction 1073742208) -> (junction 1073742210) : {
      | }
  (junction 1073742210) -> (junction 1073742212)
  (junction 1073742212) -> (junction 1073742214)
  (junction 1073742214) -> (junction 1073742216) : {
      | % END_R_25
      | }
  (junction 1073742216) -> (junction 1073742221) : {
      | % START_R_28
      | }
  (junction 1073742221) -> (junction 1073742223) : {
      | }
  (junction 1073742223) -> (junction 1073742225)
  (junction 1073742225) -> (junction 1073742227) [order 1] : [(((status) == (00101)))]
  (junction 1073742225) -> (junction 1073742233) [order 2]
  (junction 1073742227) -> (junction 1073742229) : {
      | reqtable_postcondition((((PACE_CHARGE_CTRL) == (1))) && (((Z_ATR_CTRL) == (0))) && (((Z_VENT_CTRL) == (0))) && (((ATR_PACE_CTRL) == (0))) && (((VENT_PACE_CTRL) == (0))) && (((PACE_GND_CTRL) == (1))) && (((ATR_GND_CTRL) == (1))) && (((VENT_GND_CTRL) == (0))) && (((FRONTEND_CTRL) == (1))), 'R:3.2');
      |
      |
      | }
  (junction 1073742229) -> (junction 1073742231) : {
      | }
  (junction 1073742231) -> (junction 1073742233)
  (junction 1073742233) -> (junction 1073742235)
  (junction 1073742235) -> (junction 1073742237) : {
      | % END_R_28
      | }
  (junction 1073742237) -> (junction 1073742242) : {
      | % START_R_31
      | }
  (junction 1073742242) -> (junction 1073742244) : {
      | }
  (junction 1073742244) -> (junction 1073742246)
  (junction 1073742246) -> (junction 1073742248) [order 1] : [(((status) == (00110)))]
  (junction 1073742246) -> (junction 1073742254) [order 2]
  (junction 1073742248) -> (junction 1073742250) : {
      | reqtable_postcondition((((PACE_CHARGE_CTRL) == (0))) && (((Z_ATR_CTRL) == (0))) && (((Z_VENT_CTRL) == (0))) && (((ATR_PACE_CTRL) == (1))) && (((VENT_PACE_CTRL) == (0))) && (((PACE_GND_CTRL) == (1))) && (((ATR_GND_CTRL) == (0))) && (((VENT_GND_CTRL) == (0))) && (((FRONTEND_CTRL) == (1))), 'R:3.3');
      |
      |
      | }
  (junction 1073742250) -> (junction 1073742252) : {
      | }
  (junction 1073742252) -> (junction 1073742254)
  (junction 1073742254) -> (junction 1073742256)
  (junction 1073742256) -> (junction 1073742258) : {
      | % END_R_31
      | }
  (junction 1073742258) -> (junction 1073742104) : {
      | % END_R_22
      | }
  (junction 1073742104) -> (junction 1073742275) : {
      | % START_R_34
      | }
  (junction 1073742275) -> (junction 1073742277) : {
      | }
  (junction 1073742277) -> (junction 1073742279) : {
      |
      |
      | }
  (junction 1073742279) -> (junction 1073742281) : {
      | }
  (junction 1073742281) -> (junction 1073742321) : {
      | % START_R_37
      | }
  (junction 1073742321) -> (junction 1073742323) : {
      | }
  (junction 1073742323) -> (junction 1073742325)
  (junction 1073742325) -> (junction 1073742327) [order 1] : [(((status) == (00111)))]
  (junction 1073742325) -> (junction 1073742333) [order 2]
  (junction 1073742327) -> (junction 1073742329) : {
      | reqtable_postcondition((((PACE_CHARGE_CTRL) == (1))) && (((Z_ATR_CTRL) == (0))) && (((Z_VENT_CTRL) == (0))) && (((ATR_PACE_CTRL) == (0))) && (((VENT_PACE_CTRL) == (0))) && (((PACE_GND_CTRL) == (1))) && (((ATR_GND_CTRL) == (0))) && (((VENT_GND_CTRL) == (1))) && (((FRONTEND_CTRL) == (1))), 'R:4.1');
      |
      |
      | }
  (junction 1073742329) -> (junction 1073742331) : {
      | }
  (junction 1073742331) -> (junction 1073742333)
  (junction 1073742333) -> (junction 1073742335)
  (junction 1073742335) -> (junction 1073742337) : {
      | % END_R_37
      | }
  (junction 1073742337) -> (junction 1073742342) : {
      | % START_R_40
      | }
  (junction 1073742342) -> (junction 1073742344) : {
      | }
  (junction 1073742344) -> (junction 1073742346)
  (junction 1073742346) -> (junction 1073742348) [order 1] : [(((status) == (01000)))]
  (junction 1073742346) -> (junction 1073742354) [order 2]
  (junction 1073742348) -> (junction 1073742350) : {
      | reqtable_postcondition((((PACE_CHARGE_CTRL) == (1))) && (((Z_ATR_CTRL) == (0))) && (((Z_VENT_CTRL) == (0))) && (((ATR_PACE_CTRL) == (0))) && (((VENT_PACE_CTRL) == (0))) && (((PACE_GND_CTRL) == (1))) && (((ATR_GND_CTRL) == (0))) && (((VENT_GND_CTRL) == (1))) && (((FRONTEND_CTRL) == (1))), 'R:4.2');
      |
      |
      | }
  (junction 1073742350) -> (junction 1073742352) : {
      | }
  (junction 1073742352) -> (junction 1073742354)
  (junction 1073742354) -> (junction 1073742356)
  (junction 1073742356) -> (junction 1073742358) : {
      | % END_R_40
      | }
  (junction 1073742358) -> (junction 1073742363) : {
      | % START_R_43
      | }
  (junction 1073742363) -> (junction 1073742365) : {
      | }
  (junction 1073742365) -> (junction 1073742367)
  (junction 1073742367) -> (junction 1073742369) [order 1] : [(((status) == (01001)))]
  (junction 1073742367) -> (junction 1073742375) [order 2]
  (junction 1073742369) -> (junction 1073742371) : {
      | reqtable_postcondition((((PACE_CHARGE_CTRL) == (0))) && (((Z_ATR_CTRL) == (0))) && (((Z_VENT_CTRL) == (0))) && (((ATR_PACE_CTRL) == (0))) && (((VENT_PACE_CTRL) == (1))) && (((PACE_GND_CTRL) == (1))) && (((ATR_GND_CTRL) == (0))) && (((VENT_GND_CTRL) == (0))) && (((FRONTEND_CTRL) == (1))), 'R:4.3');
      |
      |
      | }
  (junction 1073742371) -> (junction 1073742373) : {
      | }
  (junction 1073742373) -> (junction 1073742375)
  (junction 1073742375) -> (junction 1073742377)
  (junction 1073742377) -> (junction 1073742379) : {
      | % END_R_43
      | }
  (junction 1073742379) -> (junction 1073742293) : {
      | % END_R_34
      | }
  (junction 1073742293) -> (junction 1073742406) : {
      | % START_R_46
      | }
  (junction 1073742406) -> (junction 1073742408) : {
      | }
  (junction 1073742408) -> (junction 1073742410) : {
      |
      |
      | }
  (junction 1073742410) -> (junction 1073742412) : {
      | }
  (junction 1073742412) -> (junction 1073742440) : {
      | % START_R_49
      | }
  (junction 1073742440) -> (junction 1073742442) : {
      | }
  (junction 1073742442) -> (junction 1073742444)
  (junction 1073742444) -> (junction 1073742446) [order 1] : [(((status) == (01010)))]
  (junction 1073742444) -> (junction 1073742452) [order 2]
  (junction 1073742446) -> (junction 1073742448) : {
      | reqtable_postcondition((((PACE_CHARGE_CTRL) == (1))) && (((Z_ATR_CTRL) == (0))) && (((Z_VENT_CTRL) == (0))) && (((ATR_PACE_CTRL) == (0))) && (((VENT_PACE_CTRL) == (0))) && (((PACE_GND_CTRL) == (1))) && (((ATR_GND_CTRL) == (1))) && (((VENT_GND_CTRL) == (0))), 'R:5.1');
      |
      |
      | }
  (junction 1073742448) -> (junction 1073742450) : {
      | }
  (junction 1073742450) -> (junction 1073742452)
  (junction 1073742452) -> (junction 1073742454)
  (junction 1073742454) -> (junction 1073742456) : {
      | % END_R_49
      | }
  (junction 1073742456) -> (junction 1073742461) : {
      | % START_R_52
      | }
  (junction 1073742461) -> (junction 1073742463) : {
      | }
  (junction 1073742463) -> (junction 1073742465)
  (junction 1073742465) -> (junction 1073742467) [order 1] : [(((status) == (01011)))]
  (junction 1073742465) -> (junction 1073742473) [order 2]
  (junction 1073742467) -> (junction 1073742469) : {
      | reqtable_postcondition((((PACE_CHARGE_CTRL) == (0))) && (((Z_ATR_CTRL) == (0))) && (((Z_VENT_CTRL) == (0))) && (((ATR_PACE_CTRL) == (1))) && (((VENT_PACE_CTRL) == (0))) && (((PACE_GND_CTRL) == (1))) && (((ATR_GND_CTRL) == (0))) && (((VENT_GND_CTRL) == (0))), 'R:5.2');
      |
      |
      | }
  (junction 1073742469) -> (junction 1073742471) : {
      | }
  (junction 1073742471) -> (junction 1073742473)
  (junction 1073742473) -> (junction 1073742475)
  (junction 1073742475) -> (junction 1073742477) : {
      | % END_R_52
      | }
  (junction 1073742477) -> (junction 1073742424) : {
      | % END_R_46
      | }
  (junction 1073742424) -> (junction 1073742494) : {
      | % START_R_55
      | }
  (junction 1073742494) -> (junction 1073742496) : {
      | }
  (junction 1073742496) -> (junction 1073742498) : {
      |
      |
      | }
  (junction 1073742498) -> (junction 1073742500) : {
      | }
  (junction 1073742500) -> (junction 1073742528) : {
      | % START_R_58
      | }
  (junction 1073742528) -> (junction 1073742530) : {
      | }
  (junction 1073742530) -> (junction 1073742532)
  (junction 1073742532) -> (junction 1073742534) [order 1] : [(((status) == (01100)))]
  (junction 1073742532) -> (junction 1073742540) [order 2]
  (junction 1073742534) -> (junction 1073742536) : {
      | reqtable_postcondition((((PACE_CHARGE_CTRL) == (1))) && (((Z_ATR_CTRL) == (0))) && (((Z_VENT_CTRL) == (0))) && (((ATR_PACE_CTRL) == (0))) && (((VENT_PACE_CTRL) == (0))) && (((PACE_GND_CTRL) == (1))) && (((ATR_GND_CTRL) == (0))) && (((VENT_GND_CTRL) == (1))), 'R:6.1');
      |
      |
      | }
  (junction 1073742536) -> (junction 1073742538) : {
      | }
  (junction 1073742538) -> (junction 1073742540)
  (junction 1073742540) -> (junction 1073742542)
  (junction 1073742542) -> (junction 1073742544) : {
      | % END_R_58
      | }
  (junction 1073742544) -> (junction 1073742549) : {
      | % START_R_61
      | }
  (junction 1073742549) -> (junction 1073742551) : {
      | }
  (junction 1073742551) -> (junction 1073742553)
  (junction 1073742553) -> (junction 1073742555) [order 1] : [(((status) == (01101)))]
  (junction 1073742553) -> (junction 1073742561) [order 2]
  (junction 1073742555) -> (junction 1073742557) : {
      | reqtable_postcondition((((PACE_CHARGE_CTRL) == (0))) && (((Z_ATR_CTRL) == (0))) && (((Z_VENT_CTRL) == (0))) && (((ATR_PACE_CTRL) == (0))) && (((VENT_PACE_CTRL) == (1))) && (((PACE_GND_CTRL) == (1))) && (((ATR_GND_CTRL) == (0))) && (((VENT_GND_CTRL) == (0))), 'R:6.2');
      |
      |
      | }
  (junction 1073742557) -> (junction 1073742559) : {
      | }
  (junction 1073742559) -> (junction 1073742561)
  (junction 1073742561) -> (junction 1073742563)
  (junction 1073742563) -> (junction 1073742565) : {
      | % END_R_61
      | }
  (junction 1073742565) -> (junction 1073742512) : {
      | % END_R_55
      | }
  (junction 1073742512) -> (junction 1073742582) : {
      | % START_R_64
      | }
  (junction 1073742582) -> (junction 1073742584) : {
      | }
  (junction 1073742584) -> (junction 1073742586) : {
      |
      |
      | }
  (junction 1073742586) -> (junction 1073742588) : {
      | }
  (junction 1073742588) -> (junction 1073742662) : {
      | % START_R_67
      | }
  (junction 1073742662) -> (junction 1073742664) : {
      | }
  (junction 1073742664) -> (junction 1073742666)
  (junction 1073742666) -> (junction 1073742668) [order 1] : [(((status) == (01110)))]
  (junction 1073742666) -> (junction 1073742674) [order 2]
  (junction 1073742668) -> (junction 1073742670) : {
      | reqtable_postcondition((((PACE_CHARGE_CTRL) == (1))) && (((Z_ATR_CTRL) == (0))) && (((Z_VENT_CTRL) == (0))) && (((ATR_PACE_CTRL) == (0))) && (((VENT_PACE_CTRL) == (0))) && (((PACE_GND_CTRL) == (1))) && (((ATR_GND_CTRL) == (1))) && (((VENT_GND_CTRL) == (0))) && (((FRONTEND_CTRL) == (1))), 'R:7.1');
      |
      |
      | }
  (junction 1073742670) -> (junction 1073742672) : {
      | }
  (junction 1073742672) -> (junction 1073742674)
  (junction 1073742674) -> (junction 1073742676)
  (junction 1073742676) -> (junction 1073742678) : {
      | % END_R_67
      | }
  (junction 1073742678) -> (junction 1073742683) : {
      | % START_R_70
      | }
  (junction 1073742683) -> (junction 1073742685) : {
      | }
  (junction 1073742685) -> (junction 1073742687)
  (junction 1073742687) -> (junction 1073742689) [order 1] : [(((status) == (01111)))]
  (junction 1073742687) -> (junction 1073742695) [order 2]
  (junction 1073742689) -> (junction 1073742691) : {
      | reqtable_postcondition((((PACE_CHARGE_CTRL) == (1))) && (((Z_ATR_CTRL) == (0))) && (((Z_VENT_CTRL) == (0))) && (((ATR_PACE_CTRL) == (0))) && (((VENT_PACE_CTRL) == (0))) && (((PACE_GND_CTRL) == (1))) && (((ATR_GND_CTRL) == (1))) && (((VENT_GND_CTRL) == (0))) && (((FRONTEND_CTRL) == (1))), 'R:7.2');
      |
      |
      | }
  (junction 1073742691) -> (junction 1073742693) : {
      | }
  (junction 1073742693) -> (junction 1073742695)
  (junction 1073742695) -> (junction 1073742697)
  (junction 1073742697) -> (junction 1073742699) : {
      | % END_R_70
      | }
  (junction 1073742699) -> (junction 1073742704) : {
      | % START_R_73
      | }
  (junction 1073742704) -> (junction 1073742706) : {
      | }
  (junction 1073742706) -> (junction 1073742708)
  (junction 1073742708) -> (junction 1073742710) [order 1] : [(((status) == (10000)))]
  (junction 1073742708) -> (junction 1073742716) [order 2]
  (junction 1073742710) -> (junction 1073742712) : {
      | reqtable_postcondition((((PACE_CHARGE_CTRL) == (0))) && (((Z_ATR_CTRL) == (0))) && (((Z_VENT_CTRL) == (0))) && (((ATR_PACE_CTRL) == (1))) && (((VENT_PACE_CTRL) == (0))) && (((PACE_GND_CTRL) == (1))) && (((ATR_GND_CTRL) == (0))) && (((VENT_GND_CTRL) == (0))) && (((FRONTEND_CTRL) == (1))), 'R:7.3');
      |
      |
      | }
  (junction 1073742712) -> (junction 1073742714) : {
      | }
  (junction 1073742714) -> (junction 1073742716)
  (junction 1073742716) -> (junction 1073742718)
  (junction 1073742718) -> (junction 1073742720) : {
      | % END_R_73
      | }
  (junction 1073742720) -> (junction 1073742600) : {
      | % END_R_64
      | }
  (junction 1073742600) -> (junction 1073742737) : {
      | % START_R_76
      | }
  (junction 1073742737) -> (junction 1073742739) : {
      | }
  (junction 1073742739) -> (junction 1073742741) : {
      |
      |
      | }
  (junction 1073742741) -> (junction 1073742743) : {
      | }
  (junction 1073742743) -> (junction 1073742783) : {
      | % START_R_79
      | }
  (junction 1073742783) -> (junction 1073742785) : {
      | }
  (junction 1073742785) -> (junction 1073742787)
  (junction 1073742787) -> (junction 1073742789) [order 1] : [(((status) == (10001)))]
  (junction 1073742787) -> (junction 1073742795) [order 2]
  (junction 1073742789) -> (junction 1073742791) : {
      | reqtable_postcondition((((PACE_CHARGE_CTRL) == (1))) && (((Z_ATR_CTRL) == (0))) && (((Z_VENT_CTRL) == (0))) && (((ATR_PACE_CTRL) == (0))) && (((VENT_PACE_CTRL) == (0))) && (((PACE_GND_CTRL) == (1))) && (((ATR_GND_CTRL) == (0))) && (((VENT_GND_CTRL) == (1))) && (((FRONTEND_CTRL) == (1))), 'R:8.1');
      |
      |
      | }
  (junction 1073742791) -> (junction 1073742793) : {
      | }
  (junction 1073742793) -> (junction 1073742795)
  (junction 1073742795) -> (junction 1073742797)
  (junction 1073742797) -> (junction 1073742799) : {
      | % END_R_79
      | }
  (junction 1073742799) -> (junction 1073742804) : {
      | % START_R_82
      | }
  (junction 1073742804) -> (junction 1073742806) : {
      | }
  (junction 1073742806) -> (junction 1073742808)
  (junction 1073742808) -> (junction 1073742810) [order 1] : [(((status) == (10010)))]
  (junction 1073742808) -> (junction 1073742816) [order 2]
  (junction 1073742810) -> (junction 1073742812) : {
      | reqtable_postcondition((((PACE_CHARGE_CTRL) == (1))) && (((Z_ATR_CTRL) == (0))) && (((Z_VENT_CTRL) == (0))) && (((ATR_PACE_CTRL) == (0))) && (((VENT_PACE_CTRL) == (0))) && (((PACE_GND_CTRL) == (1))) && (((ATR_GND_CTRL) == (0))) && (((VENT_GND_CTRL) == (1))) && (((FRONTEND_CTRL) == (1))), 'R:8.2');
      |
      |
      | }
  (junction 1073742812) -> (junction 1073742814) : {
      | }
  (junction 1073742814) -> (junction 1073742816)
  (junction 1073742816) -> (junction 1073742818)
  (junction 1073742818) -> (junction 1073742820) : {
      | % END_R_82
      | }
  (junction 1073742820) -> (junction 1073742825) : {
      | % START_R_85
      | }
  (junction 1073742825) -> (junction 1073742827) : {
      | }
  (junction 1073742827) -> (junction 1073742829)
  (junction 1073742829) -> (junction 1073742831) [order 1] : [(((status) == (10011)))]
  (junction 1073742829) -> (junction 1073742837) [order 2]
  (junction 1073742831) -> (junction 1073742833) : {
      | reqtable_postcondition((((PACE_CHARGE_CTRL) == (0))) && (((Z_ATR_CTRL) == (0))) && (((Z_VENT_CTRL) == (0))) && (((ATR_PACE_CTRL) == (0))) && (((VENT_PACE_CTRL) == (1))) && (((PACE_GND_CTRL) == (1))) && (((ATR_GND_CTRL) == (0))) && (((VENT_GND_CTRL) == (0))) && (((FRONTEND_CTRL) == (1))), 'R:8.3');
      |
      |
      | }
  (junction 1073742833) -> (junction 1073742835) : {
      | }
  (junction 1073742835) -> (junction 1073742837)
  (junction 1073742837) -> (junction 1073742839)
  (junction 1073742839) -> (junction 1073742841) : {
      | % END_R_85
      | }
  (junction 1073742841) -> (junction 1073742755) : {
      | % END_R_76
      | }
  data: ATR_GND_CTRL input; ATR_PACE_CTRL input; VENT_GND_CTRL input; VENT_PACE_CTRL input; Z_ATR_CTRL input; Z_VENT_CTRL input; FRONTEND_CTRL input; PACE_GND_CTRL input; PACE_CHARGE_CTRL input; status input
